simulink model "single_phase_full_wave_rectifire"  (R2024a)
settings: Solver=VariableStepAuto  StartTime=0.0  StopTime=0.1  RelTol=1e-3
libraries: spsDiodeLib x4, spsRMSLib x4, spsCurrentMeasurementLib x2, spsMeanLib x2, spsVoltageMeasurementLib x2, spsACVoltageSourceLib x1, spsSeriesRLCBranchLib x1, sps_lib x1
settings Model: Creator=Asus  LastModifiedBy=Asus

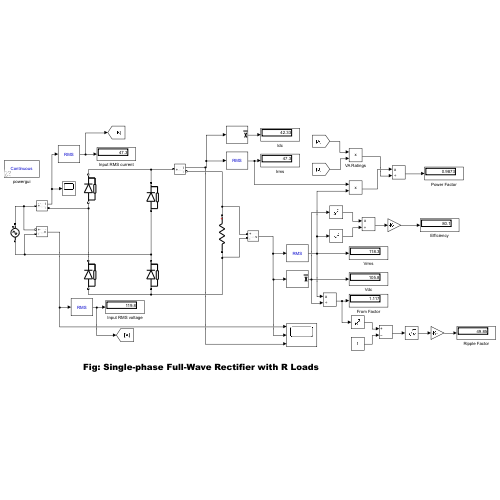
[thumbnail: Simulink's stored preview of the top-level diagram]
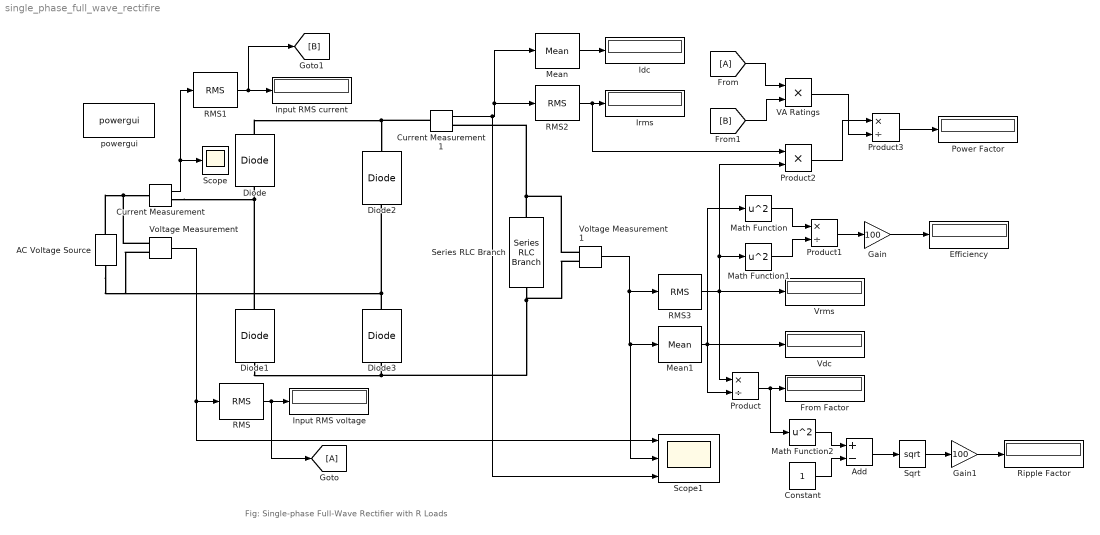
== system single_phase_full_wave_rectifire ==
  note: Fig: Single-phase Full-Wave Rectifier with R Loads
  AC Voltage Source : spsACVoltageSourceLib/AC Voltage Source  Amplitude=120*sqrt(2)  Phase=0  Frequency=60  SampleTime=0  Measurements=None  BusType=swing  Pref=10e3  Qref=0  Qmin=-inf  Qmax=+inf
  Add : Sum  Inputs=+-
  Constant : Constant
  Current Measurement : spsCurrentMeasurementLib/Current Measurement  PhasorSimulation=off  OutputType=Complex  PSBequivalent=0
  Current Measurement1 : spsCurrentMeasurementLib/Current Measurement  PhasorSimulation=off  OutputType=Complex  PSBequivalent=0
  Diode{,1..3} (4 alike) : spsDiodeLib/Diode  Ron=0.001  Lon=0  Vf=0.8  IC=0  UseSnubber=0  Rs=500  Cs=250e-9  Measurements=off
  Efficiency : Display
  From : From
  From Factor : Display
  Gain : Gain  Gain=100
  Gain1 : Gain  Gain=100
  Goto : Goto
  Idc : Display
  Input RMS current : Display
  Input RMS voltage : Display
  Irms : Display
  Math Function : Math  Operator=square
  Math Function1 : Math  Operator=square
  Math Function2 : Math  Operator=square
  Mean : spsMeanLib/Mean  Freq=60  Vinit=0  Ts=0
  Mean1 : spsMeanLib/Mean  Freq=60  Vinit=0  Ts=0
  Power Factor : Display
  Product : Product  Inputs=*/
  Product1 : Product  Inputs=*/
  Product2 : Product
  Product3 : Product  Inputs=*/
  RMS{,1..3} (4 alike) : spsRMSLib/RMS  TrueRMS=on  Freq=60  RMSInit=120  Ts=0
  Ripple Factor : Display
  Scope : Scope
  Scope1 : Scope  NumInputPorts=3
  Series RLC Branch : spsSeriesRLCBranchLib/Series RLC Branch  LConnTagsString=__new0  RConnTagsString=__new0  BranchType=R  Resistance=2.5  Inductance=1e-3  SetiL0=off  InitialCurrent=0  Capacitance=1e-6  Setx0=off  InitialVoltage=0  Measurements=None
  Sqrt : Sqrt
  VA Ratings : Product
  Vdc : Display
  Voltage Measurement : spsVoltageMeasurementLib/Voltage Measurement  PhasorSimulation=off  OutputType=Complex  PSBequivalent=0
  Voltage Measurement1 : spsVoltageMeasurementLib/Voltage Measurement  PhasorSimulation=off  OutputType=Complex  PSBequivalent=0
  Vrms : Display
  powergui : sps_lib/powergui  Priority=1  SimulationMode=Continuous  SampleTime=50e-6  frequency=60  Iterations=50  frequencyindice=60  Pbase=100e6  ErrMax=1e-4  UnitsV=kV  UnitsW=MW  buscounter=0  FunctionMessages=off  echomessages=off  EnableUseOfTLC=off  CurrentSourceSwitches=off  DisableSnubberDevices=off  DisableRonSwitches=off  DisableVfSwitches=off  DisplayEquations=off  AutomaticDiscreteSolvers=off  SolverType=Tustin/Backward Euler (TBE)  Interpol=off  ExternalGateDelay=off  methode=off  Ts=100  x0status=blocks  SPID=on  SwTol=0  HookPort=off  NonlinearTolerance=1e-4  nMaxIteration=100  ContinueOnMaxIteration=off  RestoreLinks=warning  ResistiveCurrentMeasurement=off  Frange=[0:2:500]  Ylog=off  Xlog=on  ShowGrid=off  save=off  variable=ZData  structure=0  ZoomFFT=off  StartTime=0.0  cycles=1  DisplayStyle=1  fundamental=60  FreqAxis=off  MaxFrequency=1000  frequencyindicesteady=1  RmsSteady=1  display=off
  wires:
  RMS/1 -> Goto/1, Input RMS voltage/1
  Voltage Measurement/1 -> Scope1/1, RMS/1
  Current Measurement/1 -> RMS1/1, Scope/1
  RMS1/1 -> [B], Input RMS current/1
  Current Measurement1/1 -> Scope1/3, Mean/1, RMS2/1
  Mean/1 -> Idc/1
  RMS2/1 -> Product2/1, Irms/1
  Voltage Measurement1/1 -> Scope1/2, Mean1/1, RMS3/1
  RMS3/1 -> Product/1, Vrms/1, Product2/2, Math Function1/1
  Mean1/1 -> Product/2, Math Function/1, Vdc/1
  Product/1 -> Math Function2/1, From Factor/1
  Math Function/1 -> Product1/1
  Math Function1/1 -> Product1/2
  Product1/1 -> Gain/1
  Gain/1 -> Efficiency/1
  Math Function2/1 -> Add/1
  Constant/1 -> Add/2
  Add/1 -> Sqrt/1
  Sqrt/1 -> Gain1/1
  Gain1/1 -> Ripple Factor/1
  From/1 -> VA Ratings/1
  [B] -> VA Ratings/2
  Product2/1 -> Product3/1
  VA Ratings/1 -> Product3/2
  Product3/1 -> Power Factor/1
  connections:
  Diode1/RConn1 -- Current Measurement/RConn1 -- Diode/LConn1
  Diode/RConn1 -- Current Measurement1/LConn1 -- Diode2/RConn1
  Diode3/RConn1 -- AC Voltage Source/LConn1 -- Voltage Measurement/LConn2 -- Diode2/LConn1
  AC Voltage Source/RConn1 -- Voltage Measurement/LConn1 -- Current Measurement/LConn1
  Series RLC Branch/LConn1 -- Voltage Measurement1/LConn1 -- Current Measurement1/RConn1
  Series RLC Branch/RConn1 -- Voltage Measurement1/LConn2 -- Diode1/LConn1 -- Diode3/LConn1
